simulink model "new_control"  (R2024b)
settings: Solver=FixedStepAuto  StartTime=0.0  StopTime=inf  FixedStep=0.01  RelTol=1e-3  EnableMultiTasking=on
undefined symbols (not defined in the file or in its folder): Discrete, qbreak, Time
libraries: simulink x70, arduinolib x30, dspswit3 x13, arduinosensorlib x2, ctrlSharedLib x2
(part 4 of 4)

== matlab function new_control/IMUs/SOGI + FLL (IN PHASE + QUADRATURE COMPONENT ESTIMATION)/MATLAB Function1 ==
  settings: updateMethod=DISCRETE
function [theta, theta_quad] = SOGI_FLL( ...
    x, Ts, ...
    f_min, f_max, ...     % cadence bounds (walking/running range)
    k_sogi, k_fll, ...            % FLL adaptation speed (sensor/noise dependent)
    E_lo, E_hi)           % lock thresholds (amplitude/noise dependent)


% SOGI-FLL:
%   SOGI = Second-Order Generalized Integrator (generates in-phase + quadrature)
%   FLL  = Frequency-Locked Loop (adapts internal frequency to cadence changes)
%
% INPUTS:
%   x       : drift-removed joint angle [rad] (recommended: x = theta_raw - slowLPF(theta_raw))
%   walking : boolean gate (true when moving; false when standing)
%   Ts      : sample time [s]
%
%   f_min,f_max : [Hz] plausible cadence bounds (include running if needed)
%   k_fll       : FLL adaptation gain (higher=faster, more sensitive to noise)
%   E_lo,E_hi   : energy thresholds for confidence/lock (depends on amplitude & noise)
%
% OUTPUTS:
%   theta       : in-phase filtered signal
%   theta_quad  : quadrature signal

%% -------- Fixed “rarely changed” parameters (keep inside) --------

walking = 1.0; %walking detected

fc_f_smooth = 0.30;
% Tune only if internal frequency becomes jittery or too laggy:
%   - decrease to 0.2 for smoother (more lag)
%   - increase to 0.5 for faster (more jitter)

fc_lock = 0.50;
% Tune only if lock flickers or reacts too slowly:
%   - decrease (0.3) to reduce flicker
%   - increase (0.8–1.0) for faster start/stop response

f_init = 1.4;              % [Hz] initial guess (walking/running general default)
% Tune only if you want faster lock at startup:
%   - set near typical cadence in your trials (walk ~1–2 Hz, run ~2–3 Hz)

decay_notwalking = 0.999;   % state decay when standing
% Tune only if oscillator rings too long after stopping:
%   - faster decay: 0.995
%   - slower decay: 0.9995

epsSmall = 1e-9;            % numerical safety
% Increase only if you see NaN/Inf in extreme low-motion segments (e.g., 1e-8)

%% -------------------- Persistent states --------------------
persistent va vb w_est f_state lock_state
if isempty(va)
    va = 0; vb = 0;
    w_est = 2*pi*f_init;
    f_state = f_init;
    lock_state = 0;
end

%% -------------------- Precompute smoothing coefficients --------------------
aF    = exp(-2*pi*fc_f_smooth*Ts);
aLock = exp(-2*pi*fc_lock*Ts);

%% -------------------- Frequency bounds in rad/s --------------------
w_min = 2*pi*f_min;
w_max = 2*pi*f_max;

w0 = clamp(w_est, w_min, w_max);

%% ==================== SOGI ====================
if walking
    e = x - va;

    va = va + Ts*( w0*vb + k_sogi*w0*e );
    vb = vb + Ts*( -w0*va );
else
    va = decay_notwalking*va;
    vb = decay_notwalking*vb;
    e  = 0;
end

theta = va;
theta_quad = vb;

%% ==================== Lock/confidence ====================
E = theta*theta + theta_quad*theta_quad;
lock_state = aLock*lock_state + (1-aLock)*E;

lock = clamp((lock_state - E_lo)/(E_hi - E_lo + epsSmall), 0, 1);

%% ==================== FLL ====================
if walking
    mu = (e * theta_quad) / (E + epsSmall);

    w_est = w0 + Ts * (k_fll * w0 * mu) * lock;
    w_est = clamp(w_est, w_min, w_max);

    f_raw = w_est/(2*pi);
    f_state = aF*f_state + (1-aF)*f_raw;

    w_est = 2*pi*clamp(f_state, f_min, f_max);
else
    f_state = 0.995*f_state + 0.005*f_init;
    w_est   = 2*pi*f_state;
end

end

function y = clamp(x, lo, hi)
y = min(max(x, lo), hi);
end

== stateflow chart new_control/LEFT LEG/Subsystem/Chart1 ==
  state LG
    gain=amplitude;
    sigmoid_power = sig_power;
    scale = Scale_LM;
  state DS
    gain=amplitude+0.5;
    sigmoid_power = sig_power+100;
    scale = Scale_LM-0.5;
  state AS
    gain=amplitude-2;
    sigmoid_power = sig_power+100;
    scale  = Scale_LM-0.6;
  (default) -> LG
  DS -> LG [order 1] : [class==0]
  LG -> DS [order 2] : [class==2]
  LG -> AS [order 1] : [class==1]
  AS -> LG [order 2] : [class==0]
  AS -> DS [order 1] : [class==2]
  DS -> AS [order 2] : [class==1]
  data: scale output; class input; gain output; amplitude input; sigmoid_power output; sig_power input; Scale_LM input
